simulink model "frame_6"  (Simulink 7.8)
settings: Solver=ode45  StartTime=0.0  StopTime=10.0  RelTol=1e-3
libraries: dsparch4 x3, dspsigops x1, dspsrcs4 x1
settings Model: Creator=svenhoffmann  LastModifiedBy=josef  ExtModeAutoUpdateStatusClock=off
settings DataIOCC: SignalLoggingName=sigsOut
settings DebuggingCC: SaveWithParameterizedLinksMsg=none  SignalResolutionControl=TryResolveAllWithWarning  SolverPrmCheckMsg=none  MultiTaskDSMMsg=warning  MultiTaskCondExecSysMsg=none  StrictBusMsg=None
settings HardwareCC: TargetUnknown=on
settings RTWCC: IncludeERTFirstTime=on

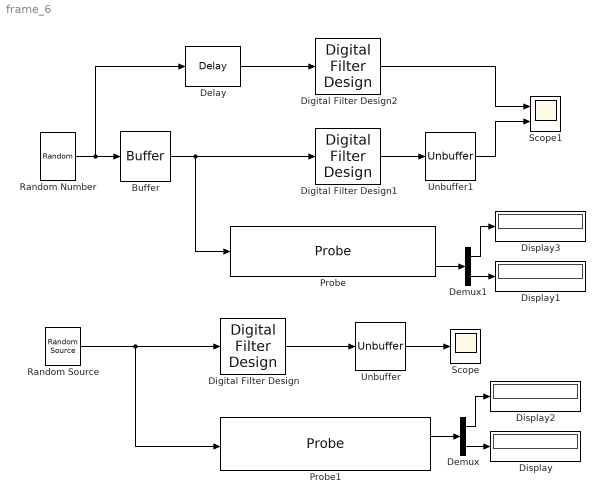
== system frame_6 ==
  Buffer : Buffer  N=1024
  Delay : dspsigops/Delay  InputProcessing=Inherited (this choice will be removed - see release notes)  dly_unit=Samples  delay=1024  ic_detail=off  dif_ic_for_ch=off  dif_ic_for_dly=off  ic=0  reset_popup=None
  Demux : Demux  Outputs=2
  Demux1 : Demux  Outputs=2
  Digital Filter Design : dsparch4/Digital Filter Design  mwdsp_browser_bugfix_var=off
  Digital Filter Design1 : dsparch4/Digital Filter Design  mwdsp_browser_bugfix_var=off
  Digital Filter Design2 : dsparch4/Digital Filter Design  mwdsp_browser_bugfix_var=off
  Display{,1..3} (4 alike) : Display
  Probe : Probe  ProbeSignalDimensions=on
  Probe1 : Probe  ProbeSignalDimensions=on
  Random Number : RandomNumber  SampleTime=1/1000
  Random Source : dspsrcs4/Random Source  SrcType=Gaussian  NormMethod=Ziggurat  CltLength=12  MinVal=0  MaxVal=1  MeanVal=0  VarVal=1  RepMode=Not repeatable  rawSeed=1  IsInherit=off  SampMode=Discrete  SampTime=1/1000  SampFrame=1024  DataType=Double  OutComplex=Real
  Scope : Scope
      settings: YMin=-1.5  YMax=1.5
  Scope1 : Scope  NumInputPorts=2
      settings: YMin=-1.5~-5  YMax=1.5~5
  Unbuffer : Unbuffer
  Unbuffer1 : Unbuffer
  wires:
  Digital Filter Design/1 -> Unbuffer/1
  Random Source/1 -> Digital Filter Design/1, Probe1/1
  Unbuffer/1 -> Scope/1
  Random Number/1 -> Buffer/1, Delay/1
  Buffer/1 -> Probe/1, Digital Filter Design1/1
  Digital Filter Design1/1 -> Unbuffer1/1
  Probe1/2 -> Demux/1
  Demux/2 -> Display/1
  Demux/1 -> Display2/1
  Demux1/2 -> Display1/1
  Demux1/1 -> Display3/1
  Probe/4 -> Demux1/1
  Digital Filter Design2/1 -> Scope1/1
  Unbuffer1/1 -> Scope1/2
  Delay/1 -> Digital Filter Design2/1
